simulink library "sig2pwm"  (R2018b)
settings: Solver=VariableStepAuto  StartTime=0.0  StopTime=10.0  RelTol=1e-3
settings Model: Creator=Robert  LastModifiedBy=Robert

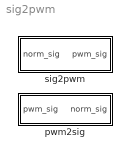
== system sig2pwm ==
  pwm2sig : Subsystem
  sig2pwm : Subsystem

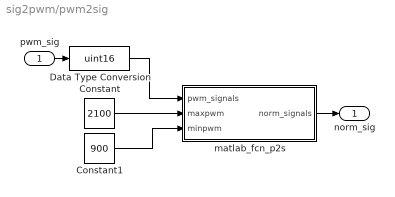
== system sig2pwm/pwm2sig ==
  pwm_sig : Inport
  Constant : Constant  Value=2100  OutDataTypeStr=uint16
  Constant1 : Constant  Value=900  OutDataTypeStr=uint16
  Data Type Conversion : DataTypeConversion  OutDataTypeStr=uint16
  matlab_fcn_p2s : MATLAB Function  TreatAsAtomicUnit=on
  norm_sig : Outport
  wires:
  matlab_fcn_p2s/1(norm_signals) -> norm_sig/1
  Constant1/1 -> matlab_fcn_p2s/3(minpwm)
  Constant/1 -> matlab_fcn_p2s/2(maxpwm)
  Data Type Conversion/1 -> matlab_fcn_p2s/1(pwm_signals)
  pwm_sig/1 -> Data Type Conversion/1

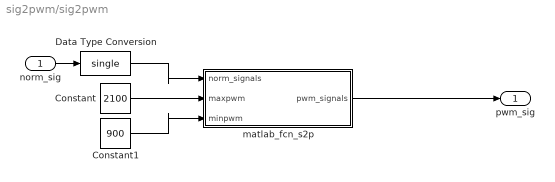
== system sig2pwm/sig2pwm ==
  norm_sig : Inport
  Constant : Constant  Value=2100  OutDataTypeStr=uint16
  Constant1 : Constant  Value=900  OutDataTypeStr=uint16
  Data Type Conversion : DataTypeConversion  OutDataTypeStr=single
  matlab_fcn_s2p : MATLAB Function  TreatAsAtomicUnit=on
  pwm_sig : Outport
  wires:
  Constant/1 -> matlab_fcn_s2p/2(maxpwm)
  matlab_fcn_s2p/1(pwm_signals) -> pwm_sig/1
  Constant1/1 -> matlab_fcn_s2p/3(minpwm)
  norm_sig/1 -> Data Type Conversion/1
  Data Type Conversion/1 -> matlab_fcn_s2p/1(norm_signals)

== matlab function sig2pwm/pwm2sig/matlab_fcn_p2s ==
  data: pwm_signals input uint16; norm_signals output single; maxpwm input uint16; minpwm input uint16
function norm_signals = pwm2signal(pwm_signals, maxpwm, minpwm)

y = single(pwm_signals);
% Shift to center
y = y-single(maxpwm);
% Range is ~1000-2000, ie +-500, but in is +-1
y = y./single(minpwm);
norm_signals = y;

== matlab function sig2pwm/matlab_fcn_s2p ==
  data: norm_signals input single; pwm_signals output uint16; maxpwm input uint16; minpwm input uint16
function pwm_signals = signal2pwm(norm_signals, maxpwm, minpwm)

pwm_signals = uint16(zeros(size(norm_signals))); % y is hard set to uint16


% Range is ~1000-2000, ie +-500, but in is +-1
norm_signals = norm_signals.*single(minpwm);
% Shift to center PWM
norm_signals = norm_signals+single(maxpwm);
pwm_signals = uint16(norm_signals);
